simulink model "simulare"  (R2023b)
settings: Solver=VariableStepAuto  StartTime=0.0  StopTime=200  RelTol=1e-3
values from neighbouring files (symbols this model uses):
  A = 1    [sysid.m]
  C = 10^-1    (= 0.1)    [sysid.m]
  D = 10^0    (= 1)    [sysid.m]
  k = place(A,B,[p1  p2  p3])    [sysid.m]
  Kd = 0.075 * Ku / Tu * D    (= 0.000143820333361)    [sysid.m]
  Ki = 1.2 * Ku / Tu * C    (= 0.000230112533377)    [sysid.m]
  Kp = Ku * 0.60    (= 0.154692)    [sysid.m]
  kr = -1*(1/(C*inv(A-B*k)*B))    [sysid.m]
undefined symbols (not defined in the file or in its folder): B, denGps, numGps
libraries: simulink x4, slpidlib x1, SignalEditorBlockLib x1
settings Model: Creator=catan  LastModifiedBy=catan

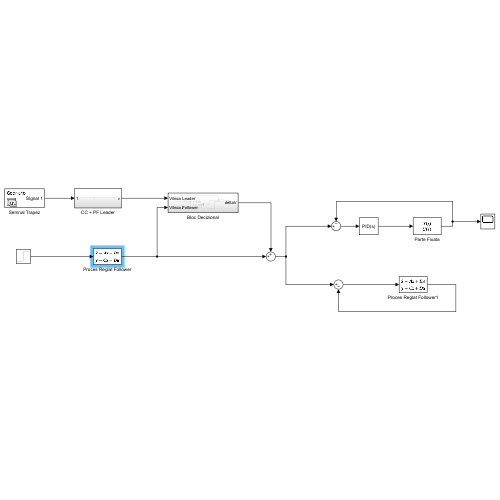
[thumbnail: Simulink's stored preview of the top-level diagram]
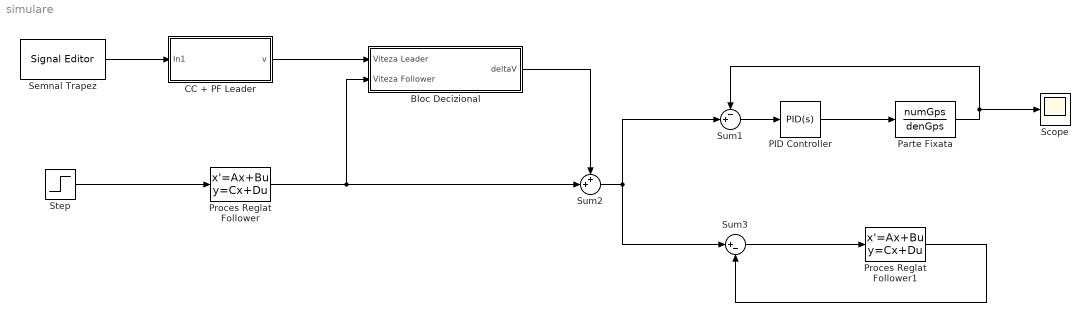
== system simulare ==
  Bloc Decizional : Subsystem
  CC + PF Leader : Subsystem
  PID Controller : slpidlib/PID Controller  Controller=PID  Form=Parallel  TimeDomain=Continuous-time  UseExternalTs=off  SampleTime=-1  IntegratorMethod=Forward Euler  FilterMethod=Forward Euler  ControllerParametersSource=internal  P=Kp  I=Ki  UseKiTs=off  D=Kd  N=5.47251376165109  UseFilter=on  TunerSelectOption=Transfer Function Based (PID Tuner App)  InitialConditionSource=internal  InitialConditionForIntegrator=0  InitialConditionForFilter=0  DifferentiatorICPrevScaledInput=0  ExternalReset=none  TrackingMode=off  Kt=1  LimitOutput=off  SatLimitsSource=internal  UpperSaturationLimit=inf  LowerSaturationLimit=-inf  LinearizeAsGain=on  AntiWindupMode=none  Kb=1  LimitIntegrator=off  UpperIntegratorSaturationLimit=inf  LowerIntegratorSaturationLimit=-inf  POutMin=[]  POutMax=[]  IOutMin=[]  IOutMax=[]  DOutMin=[]  DOutMax=[]  NOutMin=[]  NOutMax=[]  SumOutMin=[]  SumOutMax=[]  SaturationOutMin=[]  SaturationOutMax=[]  PParamMin=[]  PParamMax=[]  IParamMin=[]  IParamMax=[]  DParamMin=[]  DParamMax=[]  NParamMin=[]  NParamMax=[]  KbParamMin=[]  KbParamMax=[]  KtParamMin=[]  KtParamMax=[]  KbOutMin=[]  KbOutMax=[]  KtOutMin=[]  KtOutMax=[]  IntegratorOutMin=[]  IntegratorOutMax=[]  FilterOutMin=[]  FilterOutMax=[]  SumI1OutMin=[]  SumI1OutMax=[]  SumI2OutMin=[]  SumI2OutMax=[]  SumI3OutMin=[]  SumI3OutMax=[]  SumI4OutMin=[]  SumI4OutMax=[]  SumDOutMin=[]  SumDOutMax=[]  DifferentiatorOutMin=[]  DifferentiatorOutMax=[]  FilterDiffOutCoefMin=[]  FilterDiffOutCoefMax=[]  ReciprocalOutMin=[]  ReciprocalOutMax=[]  SumDenOutMin=[]  SumDenOutMax=[]  SumNumOutMin=[]  SumNumOutMax=[]  DivideOutMin=[]  DivideOutMax=[]  UdiffTsProdOutMin=[]  UdiffTsProdOutMax=[]  NTsProdOutMin=[]  NTsProdOutMax=[]  UintegralTsProdOutMin=[]  UintegralTsProdOutMax=[]  UngainTsProdOutMin=[]  UngainTsProdOutMax=[]  ClampingZeroOutDataTypeStr=Inherit: Inherit via back propagation  ClampingZeroOutMin=[]  ClampingZeroOutMax=[]  FilterDenConstantOutDataTypeStr=Inherit: Inherit via back propagation  FilterDenConstantOutMin=[]  FilterDenConstantOutMax=[]  PCopyOutDataTypeStr=Inherit: Inherit via back propagation  PCopyOutMin=[]  PCopyOutMax=[]  NCopyOutDataTypeStr=Inherit: Inherit via back propagation  NCopyOutMin=[]  NCopyOutMax=[]  IntegratorContinuousStateAttributes=''  IntegratorStateMustResolveToSignalObject=off  IntegratorRTWStateStorageClass=Auto  FilterContinuousStateAttributes=''  FilterStateMustResolveToSignalObject=off  FilterRTWStateStorageClass=Auto  ParallelPVariant=InternalParameters  IdealPVariant=Disabled  IVariant=InternalParameters  DVariant=InternalParameters  IntegratorVariant=Continuous  SatVariant=Disabled  AWVariant=Passthrough  PCopyVariant=Disabled  TRVariant=Disabled  FdbkBlocksVariant=Forward  IdealPFdbkVariant=Disabled  SatFdbkVariant=Disabled  DerivativeFilterVariant=ContFilter  NVariant=InternalParameters  NCopyVariant=Disabled  FilterICVariant=InternalICsFilter  IntegratorICVariant=InternalICs  ExternalResetVariant=Disabled  TRSumVariant=Passthrough  SumFdbkVariant=Disabled  SumVariant=Sum_PID  TsampFilterVariant=InternalTs  TsampNgainVariant=Passthrough  TsampIntegralVariant=Disabled_SignalSpec  ExternalSaturationOutDataTypeStr=Inherit: Same as second input
  Parte Fixata : TransferFcn  Numerator=numGps  Denominator=denGps
  Proces Reglat Follower : StateSpace  A=A - B * k  B=B * kr  C="C -  D * k"  D=D * kr  InitialCondition=0
  Proces Reglat Follower1 : StateSpace  A=A - B * k  B=B * kr  C="C -  D * k"  D=D * kr  InitialCondition=0
  Scope : Scope
  Semnal Trapez : SignalEditorBlockLib/Signal Editor  FileName=C:\Users\catan\OneDrive\Documente\semnal.mat  ActiveScenario=Scenario  ActiveSignal=Signal 1  IsBus=off  OutputBusObjectStr=Bus: BusObject  SampleTime=0  Interpolate=off  ZeroCross=off  OutputAfterFinalValue=Setting to zero  Unit=inherit  PreserveSignalName=on  ApplySigPropsToAllScenarios=on  ApplySigPropsToAllSignals=off
  Step : Step  Time=20  After=60  SampleTime=0
  Sum1 : Sum  Inputs=-+|
  Sum2 : Sum  Inputs=++|
  Sum3 : Sum  Inputs=|+-
  wires:
  Step/1 -> Proces Reglat Follower/1
  Sum1/1 -> PID Controller/1
  Semnal Trapez/1 -> CC + PF Leader/1(In1)
  CC + PF Leader/1(v) -> Bloc Decizional/1(Viteza Leader)
  PID Controller/1 -> Parte Fixata/1
  Proces Reglat Follower/1 -> Sum2/2, Bloc Decizional/2(Viteza Follower)
  Bloc Decizional/1(" deltaV") -> Sum2/1
  Proces Reglat Follower1/1 -> Sum3/2
  Sum3/1 -> Proces Reglat Follower1/1
  Sum2/1 -> Sum1/2, Sum3/1
  Parte Fixata/1 -> Sum1/1, Scope/1

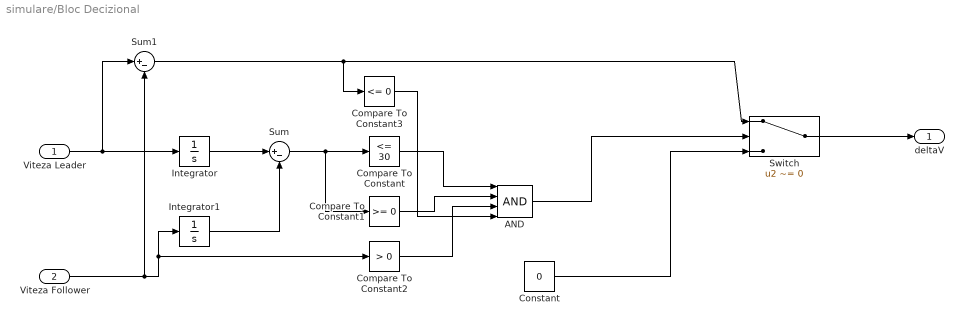
== system simulare/Bloc Decizional ==
  Viteza Leader : Inport
  Viteza Follower : Inport  Port=2
  AND : Logic  Inputs=4  IconShape=distinctive  AllPortsSameDT=off  OutDataTypeStr=boolean
  Compare To Constant : simulink/Logic and Bit Operations/Compare To Constant  relop=<=  const=30  OutDataTypeStr=boolean
  Compare To Constant1 : simulink/Logic and Bit Operations/Compare To Constant  relop=>=  const=0  OutDataTypeStr=boolean
  Compare To Constant2 : simulink/Logic and Bit Operations/Compare To Constant  relop=>  const=0  OutDataTypeStr=boolean
  Compare To Constant3 : simulink/Logic and Bit Operations/Compare To Constant  relop=<=  const=0  OutDataTypeStr=boolean
  Constant : Constant  Value=0
  Integrator : Integrator
  Integrator1 : Integrator
  Sum : Sum  Inputs=|+-
  Sum1 : Sum  Inputs=|+-
  Switch : Switch  Criteria=u2 ~= 0  SaturateOnIntegerOverflow=off  InputSameDT=off
  " deltaV" : Outport
  wires:
  Integrator/1 -> Sum/1
  Viteza Leader/1 -> Sum1/1, Integrator/1
  Switch/1 -> " deltaV"/1
  Sum/1 -> Compare To Constant1/1, Compare To Constant/1
  Integrator1/1 -> Sum/2
  Viteza Follower/1 -> Compare To Constant2/1, Integrator1/1, Sum1/2
  Compare To Constant/1 -> AND/1
  Compare To Constant1/1 -> AND/2
  AND/1 -> Switch/2
  Compare To Constant2/1 -> AND/3
  Sum1/1 -> Compare To Constant3/1, Switch/1
  Compare To Constant3/1 -> AND/4
  Constant/1 -> Switch/3

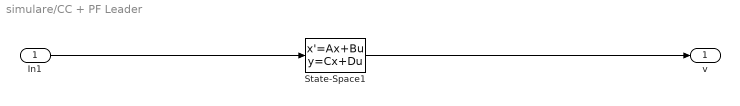
== system simulare/CC + PF Leader ==
  In1 : Inport
  State-Space1 : StateSpace  A=A - B * k  B=B * kr  C="C -  D * k"  D=D * kr  InitialCondition=0
  v : Outport
  wires:
  In1/1 -> State-Space1/1
  State-Space1/1 -> v/1
